simulink model "plosk_riskan"  (R2022b)
settings: Solver=VariableStepAuto  StartTime=0.0  StopTime=10  RelTol=1e-3
values from neighbouring files (symbols this model uses):
  k_omegay = 2.8172    [NA_ZACHET.m]    (also in Param_opt_plosk_raazv.m = x(1); obl_ust.m)
  k_psi = 9.0425    [NA_ZACHET.m]    (also in Param_opt_plosk_raazv.m = x(2); obl_ust.m)
  kzi_pr = 0.707    [NA_ZACHET.m]    (also in Param_opt_plosk_raazv.m = sqrt(2)/2; obl_ust.m)
  M_y_b = -3    [NA_ZACHET.m]    (also in Param_opt_plosk_raazv.m; obl_ust.m)
  M_y_omy = -0.2    [NA_ZACHET.m]    (also in Param_opt_plosk_raazv.m; obl_ust.m)
  M_y_sigmn = -2.5    [NA_ZACHET.m]    (also in Param_opt_plosk_raazv.m; obl_ust.m)
  om_pr = 20    [NA_ZACHET.m]    (also in Param_opt_plosk_raazv.m; obl_ust.m)
  Zb = -0.2    [NA_ZACHET.m]    (also in Param_opt_plosk_raazv.m; obl_ust.m)
libraries: checkpacklib x1
settings Model: Creator=79251  LastModifiedBy=79251

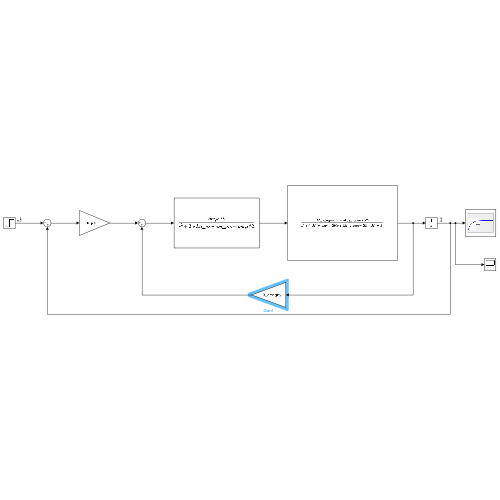
[thumbnail: Simulink's stored preview of the top-level diagram]
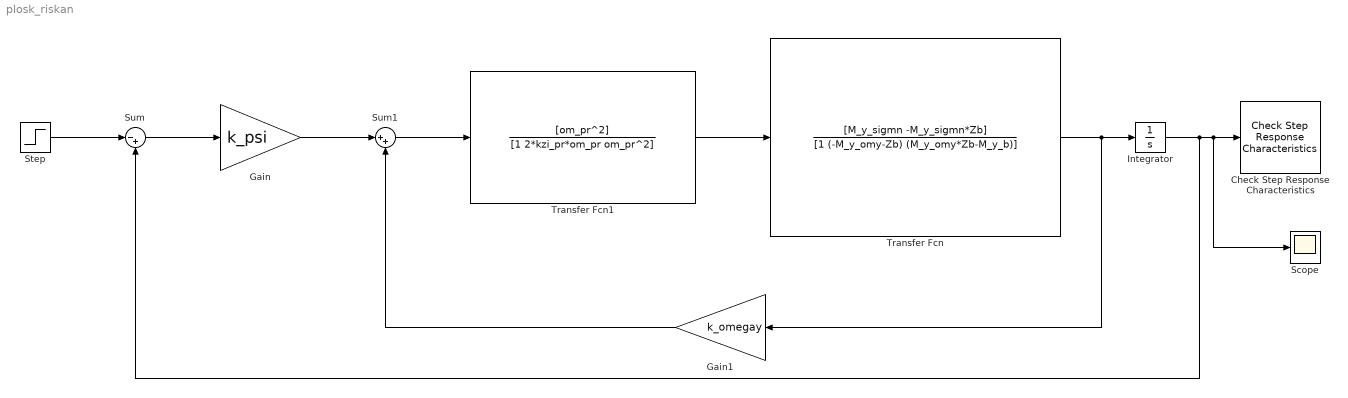
== system plosk_riskan ==
  Check Step Response Characteristics : checkpacklib/Check Step Response  Characteristics  InstantiateOnLoad=on  enabled=on  stopWhenAssertionFail=off  export=off  ViewDlgPos=[]  OpenViewOnLoad=off  LaunchViewOnOpen=off  TimeUnits=seconds  EnableStepResponseBound=on  InitialValue=0  FinalValue=1  StepTime=0  RiseTime=2  PercentRise=50  SettlingTime=3.5  PercentSettling=5  PercentOvershoot=5  PercentUndershoot=5
      settings: LibrarySourceBlock=|
      | sdolib/Model Verification/Check Step Response
      | Characteristics
  Gain : Gain  Gain=k_psi
  Gain1 : Gain  Gain=k_omegay
  Integrator : Integrator
  Scope : Scope
  Step : Step  Time=0  SampleTime=0
  Sum : Sum  Inputs=|-+
  Sum1 : Sum  Inputs=|++
  Transfer Fcn : TransferFcn  Numerator=[M_y_sigmn -M_y_sigmn*Zb]  Denominator=[1 (-M_y_omy-Zb) (M_y_omy*Zb-M_y_b)]
  Transfer Fcn1 : TransferFcn  Numerator=[om_pr^2]  Denominator=[1 2*kzi_pr*om_pr om_pr^2]
  wires:
  Sum1/1 -> Transfer Fcn1/1
  Transfer Fcn/1 -> Gain1/1, Integrator/1
  Gain/1 -> Sum1/1
  Sum/1 -> Gain/1
  Step/1 -> Sum/1
  Gain1/1 -> Sum1/2
  Integrator/1 -> Scope/1, Check Step Response Characteristics/1, Sum/2
  Transfer Fcn1/1 -> Transfer Fcn/1
